simulink model "pdmRecipPump"  (R2025b)
settings: Solver=VariableStepAuto  StartTime=0.0  StopTime=2  RelTol=1e-3  EnableMultiTasking=on
values from neighbouring files (symbols this model uses):
  s = load(dataFile)    [run_0.m]    (also in run_1.m; run_2.m; run_3.m; run_4.m)
undefined symbols (not defined in the file or in its folder): bearing_fault_frict_WKSP, bearing_visc_frict_WKSP, noise_seed_offset_WKSP, smiData, TRP_Par, X, Y, Z
libraries: sm_lib x41, fl_lib x23, nesl_utility x9, simulink x7, SimscapeFluids_lib x4, sm_pump_triplex_lib x3, ee_lib x2, Mech_Hydro_Elec_Multibody_Lib x1
(part 1 of 2)
CloseFcn:
  | try,close(h1_sm_pump_triplex),end
  | clear h1_sm_pump_triplex
  | try,close(h2_sm_pump_triplex),end
  | clear h2_sm_pump_triplex
  | try,close(h3_sm_pump_triplex),end
  | clear h3_sm_pump_triplex
  | try,close(h4_sm_pump_triplex),end
  | clear h4_sm_pump_triplex
  | try,close(h5_sm_pump_triplex),end
  | clear h5_sm_pump_triplex
  | try,close(h6_sm_pump_triplex),end
  | clear h6_sm_pump_triplex
  | try,close(h7_sm_pump_triplex),end
  | clear h7_sm_pump_triplex
  | 
  | clear simlog_sm_pump_triplex
  | clear logsout_sm_pump_triplex
Description:
  | Triplex Pump with Faults
settings Model: SimulationMode=accelerator  Creator=The MathWorks, Inc.  LastModifiedBy=The MathWorks, Inc.
settings SolverCC: MaxConsecutiveMinStep=10  AlgebraicLoopSolver=TrustRegion
settings DataIOCC: InitialState=sm_pump_triplex_xFinal_steady_no_fault  LimitDataPoints=on  MaxDataPoints=10000  SignalLoggingName=logsout_sm_pump_triplex
settings OptimizationCC: LifeSpan=inf
settings DebuggingCC: AlgebraicLoopMsg=error  UnconnectedInputMsg=warning  UnconnectedOutputMsg=warning  UnconnectedLineMsg=warning  AllowSymbolicDim=off  SFUnexpectedBacktrackingDiag=warning  SFNoUnconditionalDefaultTransitionDiag=warning  SFExecutionAtInitializationDiag=none  ArithmeticOperatorsInVariantConditions=warning
settings ModelReferenceCC: EnableRefExpFcnMdlSchedulingChecks=on
settings SFSimCC: SimUseLocalCustomCode=off  CustomCodeUndefinedFunction=UseInterfaceOnly
settings RTWCC: RTWUseLocalCustomCode=off  GPUComputeCapability=3.5
settings CodeAppCC: StateflowObjectComments=on
settings GRTTargetCC: TargetLangStandard=C89/C90 (ANSI)
settings ConfigComp: CovMetricSettings=dw  CovSaveCumulativeToWorkspaceVar=on  CovSaveSingleToWorkspaceVar=on  CovExternalEMLEnable=off  CovSFcnEnable=off
settings SimscapeCC: SimscapeNominalValues="[{\"value\":\"10\",\"unit\":\"V\"},{\"value\":\"1\",\"unit\":\"A\"},{\"value\":\"10\",\"unit\":\"N*m\"},{\"value\":\"10\",\"unit\":\"bar\"},{\"value\":\"100\",\"unit\":\"kJ/kg\"},{\"value\":\"1\",\"unit\":\"kW\"},{\"value\":\"300\",\"unit\":\"K\"},{\"value\":\"100\",\"unit\":\"cm^3/s\"},{\"value\":\"1\",\"unit\":\"kN\"},{\"value\":\"1\",\"unit\":\"g/cm^3\"},{\"value\":\"1\",\"unit\":\"l\"},{\"value\":\"1\",\"unit\":\"cm^2\"},{\"value\":\"60\",\"unit\":\"Hz\"}]"  SimscapeLogType=all  SimscapeLogSimulationStatistics=on  SimscapeLogName=simlog_sm_pump_triplex  SimscapeLogDataHistory=20000.0  SimscapeOperatingPoint=sm_pump_triplex_op_steady_no_fault
settings ConfigurationSet: Description=SimMechanics 2G
settings DiagnosticsConfigSet: SimMechanicsUnsatisfiedHighPriorityTargets=none
settings ExplorerConfigSet: SimMechanicsOpenEditorOnUpdate=off  InternalSimMechanicsExplorerSettings="<ExplorerConfiguration><canonicalview>default</canonicalview><AnimationSetting><BasePlaybackSpeed>1.0</BasePlaybackSpeed><PlaybackSpeedFactor>0.0625</PlaybackSpeedFactor></AnimationSetting><TilePanel><TileInfo><Tiles Columns=\"1\" Count=\"1\" Rows=\"1\"><Column Weight=\"1\"/><Row Weight=\"1\"/><Tile Height=\"1\" Width=\"1\" X=\"0\" Y=\"0\"/></Tiles></TileInfo><SceneInfo><SceneViewer><BGColor><R>1</R><G>1</G><B>1</B></BGColor><Camera><DoPerspective>off</DoPerspective><Position><X>0.7191096199114555</X><Y>0.503364840615347475</Y><Z>-0.352088882323819574</Z></Position><Center><X>-0.0103509884654966189</X><Y>-0.00162371159480596133</Y><Z>0.10929358696063457</Z></Center><Up><X>-0.420672049294932404</X><Y>0.863070110116374023</Y><Z>0.279544293387851028</Z></Up><ViewLimDist>1</ViewLimDist><YLim>0.161872532968254601</YLim><XLim>0.255851100680109855</XLim></Camera></SceneViewer></SceneInfo></TilePanel><MechEditorPanel><Cameras/><GfxPanelCameraMap/><VideoCreator><PlaybackSpeedRatio>1.0</PlaybackSpeedRatio><FrameRate>30</FrameRate><VideoFormat>Motion JPEG AVI</VideoFormat><FrameSize>auto</FrameSize></VideoCreator></MechEditorPanel></ExplorerConfiguration>"

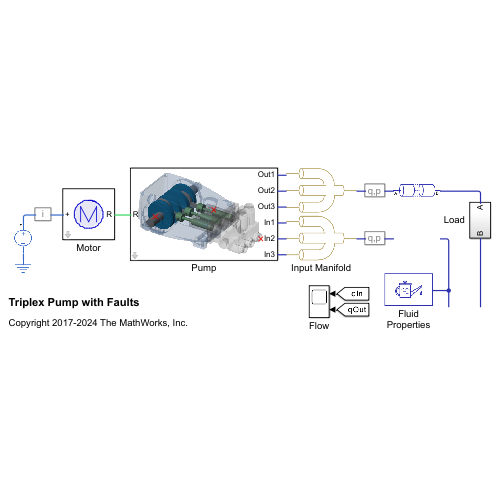
[thumbnail: Simulink's stored preview of the top-level diagram]
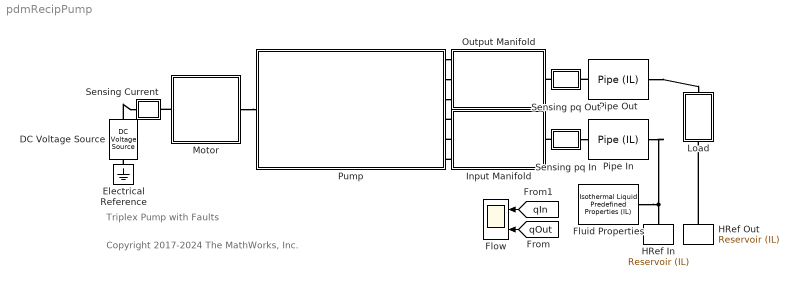
== system pdmRecipPump ==
  note: Copyright 2017-2024 The MathWorks, Inc.
  note: Triplex Pump with Faults
  DC Voltage Source : ee_lib/Additional Components/SPICE Sources/DC Voltage Source  DC=24 V
  Electrical Reference : fl_lib/Electrical/Electrical Elements/Electrical Reference
  Flow : Scope  NumInputPorts=2
      settings: ActiveDisplayYMinimum=-5.41174  ActiveDisplayYMaximum=48.70569
  Fluid Properties : SimscapeFluids_lib/Isothermal Liquid/Utilities/Isothermal Liquid Predefined Properties (IL)  fluid_list=13  concentration_param_EG=fluids.isothermal_liquid.utilities.enum.isothermal_liquid_concentration.volume_fraction  concentration_param_PG=fluids.isothermal_liquid.utilities.enum.isothermal_liquid_concentration.volume_fraction  c_mass_SW=3.5e-3  c_mass_EG=0.1  c_mass_PG=0.1  c_mass_GL=0.1  c_vol_EG=0.1  c_vol_PG=0.1  beta_L_atm_EG=2.1791 GPa  beta_L_atm_PG=2.1791 GPa  beta_L_atm_GL=2.1791 GPa  p_min_EG=0.01 MPa  p_min_PG=0.01 MPa  p_min_GL=0.01 MPa  T=60 degC  derate_coeff=1  p_atm=0.101325 MPa  properties_range_check=simscape.enum.assert.action.error  air_fraction=0.005  polytropic_index=1.0  rho_g_atm=851.6 kg/m^3  air_dissolution_model=false  p_crit=3 MPa
      settings: LibrarySourceBlock=SimscapeFluids_lib/Isothermal Liquid/Utilities/Isothermal Liquid Predefined Properties (IL)  InternalSimscapePortConfiguration="{\"Bottom\":[],\"Left\":[],\"Right\":[{\"id\":\"A\",\"label\":\"\",\"type\":\"foundation.isothermal_liquid.isothermal_liquid\"}],\"Top\":[]}"
  HRef In : fl_lib/Isothermal Liquid/Elements/Reservoir (IL)  reservoir_type=foundation.enum.constant_controlled.constant  pressure_spec=foundation.enum.pressure_spec.atmospheric  reservoir_pressure=0.101325 MPa
  HRef Out : fl_lib/Isothermal Liquid/Elements/Reservoir (IL)  reservoir_type=foundation.enum.constant_controlled.constant  pressure_spec=foundation.enum.pressure_spec.atmospheric  reservoir_pressure=0.101325 MPa
  Input Manifold : Subsystem
      mask Display: image('sm_pump_triplex_Manifold_IMAGE.png');
  Load : Subsystem
  Motor : Subsystem  Tag=PublishSubsystem  VariantControl=Electric  mask(Motor and Motor Driver){winding_fault_enable=Off}
      mask prompts: winding_fault_enable "Winding Fault"
      mask help: Model abstracts the torque-speed behavior of the combined motor and motor driver. Electric and control parameters are specified on blocks within the subsystem. The winding fault modelsa broken winding. When enabled, motor torque is set to 0 when the shaft angle is between 240 and 360 degrees (one-third of a shaft rotation).
      mask TypeOptions winding_fault_enable: Off | On
      mask Display:
      | % Circle
      | patch(sin(0:0.1:2.2*pi)*0.80,cos(0:0.1:2.2*pi)*0.80,[0.9 0.9 0.97]);
      | color('blue');
      | plot(sin(0:0.1:2.2*pi)*0.9,cos(0:0.1:2.2*pi)*0.9);
      | 
      | % 'M'
      | plot([0.5 0.5],[-0.5 0.5]);
      | plot([-0.5 -0.5],[-0.5 0.5]);
      | plot([0.5 0],[0.5 -0.5]);
      | plot([-0.5 0],[0.5 -0.5]);
      | 
      | color('red');
      | if(strcmp(get_param(gcb,'winding_fault_enable'),'On'))
      |     plot([0.85 0.6],[1.1 0.9])
      |     plot([0.6 0.85],[1.1 0.9])
      | end
      | 
      | % Plot points to set plot range
      | color('white');plot(1.6,1.6);plot(-1.6,-1.6)
      | color('black');
  Output Manifold : Subsystem
      mask Display: image('sm_pump_triplex_Manifold_IMAGE.png');
  Pipe In : SimscapeFluids_lib/Isothermal Liquid/Pipes & Fittings/Pipe (IL)  dynamic_compressibility=true  inertia=false  num_segments=1  pipe_length=5 m  cross_section_geometry=fluids.isothermal_liquid.pipes_fittings.enum.cross_section_geometry.circular  pipe_diameter=0.03 m  pipe_inner_diameter=0.05 m  pipe_outer_diameter=0.1 m  pipe_width=0.1 m  pipe_height=0.1 m  pipe_major_axis=0.1 m  pipe_minor_axis=0.05 m  pipe_side=0.1 m  pipe_angle=30 deg  pipe_area=1e-4 m^2  Dh=1.12e-2 m  elevation_spec=foundation.enum.constant_variable.constant  elevation_gain=0 m  gravity_spec=foundation.enum.constant_variable.constant  g=9.81 m/s^2  pressure_loss_spec=fluids.isothermal_liquid.pipes_fittings.enum.pressure_loss_spec.haaland  mdot_nominal=[.1, 1] kg/s  p_diff_nominal=[.001, .01] MPa  mdot_threshold=1e-6 kg/s  local_pressure_loss_spec=fluids.isothermal_liquid.pipes_fittings.enum.local_loss_spec.aggregate_length  length_add=1 m  loss_coefficient=0.1  roughness_spec=fluids.isothermal_liquid.pipes_fittings.enum.roughness_spec.custom  roughness=15e-6 m  Re_friction_TLU=[400, 1000, 1500, 3000, 4000, 6000, 10000, 20000, 40000, 60000, 100000, 100000000]  friction_factor_TLU=[.264, .112, .071, .0417, .0387, .0268, .025, .0232, .0226, .022, .0214, .0214]  Re_lam=2000  Re_tur=4000  shape_factor=64  pipe_wall_spec=fluids.isothermal_liquid.pipes_fittings.enum.wall_spec.rigid  vol_expansion_spec=fluids.isothermal_liquid.pipes_fittings.enum.vol_expansion_spec.area  area_pressure_gain=1e-6 m^2/MPa  static_pressure_TLU=[.1, 1] MPa  area_pressure_gain_TLU=[1e-05, 1.1e-05] m^2  material_behavior_spec=fluids.isothermal_liquid.pipes_fittings.enum.PipeMaterialBehavior.Linear  diameter_pressure_gain=2e-12 m/Pa  wall_thickness=0.05 m  elastic_modulus=69 GPa  stress_TLU=[276, 310] MPa  strain_TLU=[.004, .02]  stress_assert_action=simscape.enum.assert.action.none  stress_max=400 MPa  poisson_ratio=0.33  wall_time_constant=0.01 s  p0=0 + 101325 Pa  mdot0=0 kg/s
      settings: InternalSimscapePortConfiguration="{\"Bottom\":[],\"Left\":[{\"id\":\"A\",\"label\":\"A\",\"type\":\"foundation.isothermal_liquid.isothermal_liquid\"}],\"Right\":[{\"id\":\"B\",\"label\":\"B\",\"type\":\"foundation.isothermal_liquid.isothermal_liquid\"}],\"Top\":[]}"
  Pipe Out : SimscapeFluids_lib/Isothermal Liquid/Pipes & Fittings/Pipe (IL)  dynamic_compressibility=true  inertia=false  num_segments=1  pipe_length=5 m  cross_section_geometry=fluids.isothermal_liquid.pipes_fittings.enum.cross_section_geometry.circular  pipe_diameter=0.03 m  pipe_inner_diameter=0.05 m  pipe_outer_diameter=0.1 m  pipe_width=0.1 m  pipe_height=0.1 m  pipe_major_axis=0.1 m  pipe_minor_axis=0.05 m  pipe_side=0.1 m  pipe_angle=30 deg  pipe_area=1e-4 m^2  Dh=1.12e-2 m  elevation_spec=foundation.enum.constant_variable.constant  elevation_gain=0 m  gravity_spec=foundation.enum.constant_variable.constant  g=9.81 m/s^2  pressure_loss_spec=fluids.isothermal_liquid.pipes_fittings.enum.pressure_loss_spec.haaland  mdot_nominal=[.1, 1] kg/s  p_diff_nominal=[.001, .01] MPa  mdot_threshold=1e-6 kg/s  local_pressure_loss_spec=fluids.isothermal_liquid.pipes_fittings.enum.local_loss_spec.aggregate_length  length_add=1 m  loss_coefficient=0.1  roughness_spec=fluids.isothermal_liquid.pipes_fittings.enum.roughness_spec.custom  roughness=15e-6 m  Re_friction_TLU=[400, 1000, 1500, 3000, 4000, 6000, 10000, 20000, 40000, 60000, 100000, 100000000]  friction_factor_TLU=[.264, .112, .071, .0417, .0387, .0268, .025, .0232, .0226, .022, .0214, .0214]  Re_lam=2000  Re_tur=4000  shape_factor=64  pipe_wall_spec=fluids.isothermal_liquid.pipes_fittings.enum.wall_spec.rigid  vol_expansion_spec=fluids.isothermal_liquid.pipes_fittings.enum.vol_expansion_spec.area  area_pressure_gain=1e-6 m^2/MPa  static_pressure_TLU=[.1, 1] MPa  area_pressure_gain_TLU=[1e-05, 1.1e-05] m^2  material_behavior_spec=fluids.isothermal_liquid.pipes_fittings.enum.PipeMaterialBehavior.Linear  diameter_pressure_gain=2e-12 m/Pa  wall_thickness=0.05 m  elastic_modulus=69 GPa  stress_TLU=[276, 310] MPa  strain_TLU=[.004, .02]  stress_assert_action=simscape.enum.assert.action.none  stress_max=400 MPa  poisson_ratio=0.33  wall_time_constant=0.01 s  p0=TRP_Par.Spec.p_output + 1.01325 bar  mdot0=0 kg/s
      settings: InternalSimscapePortConfiguration="{\"Bottom\":[],\"Left\":[{\"id\":\"A\",\"label\":\"A\",\"type\":\"foundation.isothermal_liquid.isothermal_liquid\"}],\"Right\":[{\"id\":\"B\",\"label\":\"B\",\"type\":\"foundation.isothermal_liquid.isothermal_liquid\"}],\"Top\":[]}"
  Pump : Subsystem  Tag=PublishSubsystem  mask(Triplex Pump with Faults){cyl_gap_P=TRP_Par.Cylinder.gap, cyl_rad_out_P=TRP_Par.Cylinder.rad_outer, cyl_len_P=TRP_Par.Cylinder.len, cyl_stroke_P=TRP_Par.Cylinder.stroke, cyl_frict_brkway_frc_P=TRP_Par.Cylinder.Friction.BrkFrc, cyl_frict_brkway_vel_P=TRP_Par.Cylinder.Friction.BrkVel, cyl_frict_col_frc_P=TRP_Par.Cylinder.Friction.ColFrc, cyl_frict_visc_coef_P=TRP_Par.Cylinder.Friction.ViscCo, cyl_rho_P=TRP_Par.Cylinder.rho, cyl_clr_P=TRP_Par.Cylinder.clr, cyl_opc_P=TRP_Par.Cylinder.opc, plgB_len_P=TRP_Par.Plunger.len, plgB_rad_P=TRP_Par.Plunger.rad, stem_len_P=TRP_Par.Stem.len, stem_rad_P=TRP_Par.Stem.rad, pin_len_P=TRP_Par.Pin.len, pin_rad_P=TRP_Par.Pin.rad, cup_rad_out_P=TRP_Par.StemCup.rad, cup_thk_P=TRP_Par.StemCup.wall, cup_len_P=TRP_Par.StemCup.len, cup_pinOffset_P=TRP_Par.StemCup.pinOffset, plg_rho_P=TRP_Par.Plunger.rho, plg_clr_P=TRP_Par.Plunger.clr, plg_opc_P=TRP_Par.Plunger.opc, conrod_len_P=TRP_Par.ConRod.len, conrod_web_widP_P=TRP_Par.ConRod.W1, conrod_web_widC_P=TRP_Par.ConRod.W2, conrod_ringC_wid_P=TRP_Par.ConRod.R2.width, conrod_ringP_wid_P=TRP_Par.ConRod.R1.width, crank_shaft_rad_P=TRP_Par.Crank.Shaft.rad, conrod_thk_P=TRP_Par.ConRod.hei, conrod_rho_P=TRP_Par.ConRod.rho, conrod_clr_P=TRP_Par.ConRod.clr, conrod_opc_P=TRP_Par.ConRod.opc, chkv_in_maxA_P=TRP_Par.Check_Valve.In.Max_Area, chkv_out_maxA_P=TRP_Par.Check_Valve.Out.Max_Area, chkv_in_crkP_P=TRP_Par.Check_Valve.In.Crack_Pr, chkv_out_crkP_P=TRP_Par.Check_Valve.Out.Crack_Pr, chkv_in_maxOpenP_P=TRP_Par.Check_Valve.In.Max_Open_Pr, chkv_out_maxOpenP_P=TRP_Par.Check_Valve.Out.Max_Open_Pr, chkv_vis_popup_P=Off, chkv_vis_rad_in_P=TRP_Par.Check_Valve.In.Vis.rad, chkv_vis_rad_out_P=TRP_Par.Check_Valve.Out.Vis.rad, chkv_vis_clr_in_P=TRP_Par.Check_Valve.In.Vis.clr, chkv_vis_clr_out_P=TRP_Par.Check_Valve.Out.Vis.clr, shaft_rad_P=TRP_Par.Crank.Shaft.rad, shaft_len_P=TRP_Par.Crank.Shaft.len, web_rad_P=TRP_Par.Crank.Cam.rad, web_len_P=TRP_Par.Crank.Cam.wid, motor_shaft_rad_P=TRP_Par.Motor.Shaft.rad, motor_shaft_len_P=TRP_Par.Motor.Shaft.len, shaft_pos_P=TRP_Par.Crank.Shaft.pos, crank_rho_P=TRP_Par.Crank.rho, bearing_visc_frict=TRP_Par.Crank.Bearing.b, crank_clr_P=TRP_Par.Crank.Cam.clr, motor_shaft_clr_P=TRP_Par.Motor.Shaft.clr, crank_opc_P=TRP_Par.Crank.Cam.opc, crank_ax_offset=TRP_Par.Crank.axoffset, bearing_sep=TRP_Par.Crank.Bearing_sep, housing_clr=TRP_Par.Housing.clr, housing_opc=TRP_Par.Housing.opc, manifold_clr=TRP_Par.Manifold.clr, manifold_opc=TRP_Par.Manifold.opc, leak_cyl1_popup=On, Run Time, leak_cyl2_popup=Off, leak_cyl3_popup=Off, leak_cyl1_area=TRP_Par.Check_Valve.In.Max_Area*0.05, leak_cyl2_area=TRP_Par.Check_Valve.In.Max_Area*0.05, leak_cyl3_area=TRP_Par.Check_Valve.In.Max_Area*0.05, block_in_cyl1_popup=On, Run Time, block_in_cyl2_popup=Off, block_in_cyl3_popup=Off, block_in_cyl1_factor=0.5, block_in_cyl2_factor=0.5, block_in_cyl3_factor=0.5, bearing_fault_popup=On, Run Time, bearing_fault_frict=3e-4, seal_leak_vis_len_P=TRP_Par.Seal_Leak.len, seal_leak_vis_rad_P=TRP_Par.Seal_Leak.rad, seal_leak_vis_clr_P=TRP_Par.Seal_Leak.clr, inlet_obstr_len_P=TRP_Par.Manifold.Inlet.obstr.len, inlet_obstr_rad_P=TRP_Par.Manifold.Inlet.rad, inlet_obstr_clr_P=TRP_Par.Manifold.Inlet.obstr.clr, bearing_fault_vis_len=TRP_Par.Crank.Bearing_Fault.len, bearing_fault_vis_rad=TRP_Par.Crank.Bearing_Fault.rad, bearing_fault_vis_clr=TRP_Par.Crank.Bearing_Fault.clr, bearing_fault_vis_opc=0}
      mask prompts: cyl_gap_P "Gap (m)"; cyl_rad_out_P "Outer Radius (m)"; cyl_len_P "Length (m)"; cyl_stroke_P "Stroke (m)"; cyl_frict_brkway_frc_P "Breakaway Friction Force (N)"; cyl_frict_brkway_vel_P "Breakaway Friction Velocity (m/s)"; cyl_frict_col_frc_P "Coulomb Friction Force (N)"; cyl_frict_visc_coef_P "Viscous Friction Coeff (N/(m/s))"; cyl_rho_P "Density (kg/m^3)"; cyl_clr_P "Color [RGB]"; cyl_opc_P "Opacity (0-1)"; cup_rad_out_P "Outer Radius (m)"; cup_thk_P "Wall Thickness (m)"; cup_len_P "Length(m)"; cup_pinOffset_P "Pin Offset (m)"; plg_rho_P "Density (kg/m^3)"; plg_clr_P "Color [RGB]"; plg_opc_P "Opacity (0-1)"; conrod_len_P "Length, center-center (m)"; conrod_web_widP_P "Width, pin end (m)"; conrod_web_widC_P "Width, crank end (m)"; conrod_ringC_wid_P "Crank Ring Width (m)"; conrod_ringP_wid_P "Pin Ring Width (m)"; crank_shaft_rad_P "Crank Shaft Radius (m)"; conrod_thk_P "Thickness (m)"; conrod_rho_P "Density (kg/m^3)"; conrod_clr_P "Color [RGB]"; conrod_opc_P "Opacity (0-1)"; chkv_vis_popup_P "Valve Visualization"; shaft_pos_P "Crankpin Axis Offset (m)"; crank_rho_P "Density (kg/m^3)"; bearing_visc_frict "Bearing Viscous Friction (N*m/(deg/s))"; crank_clr_P "Crank Color [RGB]"; motor_shaft_clr_P "Motor Shaft Color [RGB]"; crank_opc_P "Opacity (0-1)"; crank_ax_offset "Crankshaft Axis Offset [XYZ] (m)"; bearing_sep "Bearing Separation (m)"; housing_clr "Housing Color [RGB]"; housing_opc "Housing Opacity (0-1)"; manifold_clr "Manifold Color [RGB]"; manifold_opc "Manifold Opacity (0-1)"; leak_cyl1_area "Plunger 1 Leak Area (m^2)"; leak_cyl2_area "Plunger 2 Leak Area (m^2)"; leak_cyl3_area "Plunger 3 Leak Area (m^2)"; block_in_cyl1_factor "Blocked Inlet 1: Area Factor (0-1)"; block_in_cyl2_factor "Blocked Inlet 2: Area Factor (0-1)"; block_in_cyl3_factor "Blocked Inlet 3: Area Factor (0-1)"; bearing_fault_popup "Bearing Wear"; bearing_fault_frict "Additional Friction (N*m/(deg/s))"; seal_leak_vis_len_P "Length (m)"; seal_leak_vis_rad_P "Radius (m)"; seal_leak_vis_clr_P "Color [RGB]"; inlet_obstr_len_P "Length (m)"; inlet_obstr_rad_P "Radius (m)"; inlet_obstr_clr_P "Color [RGB]"; bearing_fault_vis_len "Length (m)"; bearing_fault_vis_rad "Radius (m)"; bearing_fault_vis_clr "Color [RGB]"; bearing_fault_vis_opc "Opacity (0-1)"
      mask help: Models a triplex pump. Three hydraulic plungers are connected to a crankshaft. Hydraulic and mechanical faults can be enabled on the Faults tab.
      mask init:
      | % -- Configure Plunger Faults
      | set_param([gcb '/Plunger 1'],'leak_cyl_popup',...
      |     get_param(gcb,'leak_cyl1_popup'));
      | set_param([gcb '/Plunger 2'],'leak_cyl_popup',...
      |     get_param(gcb,'leak_cyl2_popup'));
      | set_param([gcb '/Plunger 3'],'leak_cyl_popup',...
      |     get_param(gcb,'leak_cyl3_popup'));
      | 
      | set_param([gcb '/Plunger 1'],'block_in_popup',...
      |     get_param(gcb,'block_in_cyl1_popup'));
      | set_param([gcb '/Plunger 2'],'block_in_popup',...
      |     get_param(gcb,'block_in_cyl2_popup'));
      | set_param([gcb '/Plunger 3'],'block_in_popup',...
      |     get_param(gcb,'block_in_cyl3_popup'));
      | 
      | % -- Set valve visualization
      | set_param([gcb '/Plunger 1'],'chkv_vis_popup',...
      |     get_param(gcb,'chkv_vis_popup_P'));
      | set_param([gcb '/Plunger 2'],'chkv_vis_popup',...
      |     get_param(gcb,'chkv_vis_popup_P'));
      | set_param([gcb '/Plunger 3'],'chkv_vis_popup',...
      |     get_param(gcb,'chkv_vis_popup_P'));
      | 
      | % -- Configure bearing fault
      | if(bearing_fault_popup==1)
      |     set_param([gcb '/Revolute Crank'],...
      |         'DampingCoefficient','bearing_visc_frict',...
      |         'DampingCoefficient_conf','compiletime');
      |     bearing_fault_vis_opc = 0;
      | elseif(bearing_fault_popup==2)
      |     set_param([gcb '/Revolute Crank'],...
      |         'DampingCoefficient','bearing_visc_frict+bearing_fault_frict',...
      |         'DampingCoefficient_conf','compiletime');
      |     bearing_fault_vis_opc = 1;
      | elseif(bearing_fault_popup==3)
      |     set_param([gcb '/Revolute Crank'],...
      |         'DampingCoefficient','bearing_visc_frict_WKSP+bearing_fault_frict_WKSP',...
      |         'DampingCoefficient_conf','runtime');
      |     bearing_fault_vis_opc = 1;
      | end
      mask TypeOptions chkv_vis_popup_P: Off | On
      mask TypeOptions leak_cyl1_popup: Off | On | On, Run Time
      mask Callback leak_cyl1_popup:
      | maskObj = Simulink.Mask.get(gcb);
      | leak_cyl1_area_h = maskObj.getParameter('leak_cyl1_area');
      | leak_cyl1_text_h = maskObj.getDialogControl('leak_cyl1_tune_text');
      | if (strcmp(get_param(gcb,'leak_cyl1_popup'),'Off'))
      |     leak_cyl1_area_h.Visible = 'off';
      |     leak_cyl1_text_h.Visible = 'off';
      | elseif (strcmp(get_param(gcb,'leak_cyl1_popup'),'On'))
      |     leak_cyl1_area_h.Visible = 'on';
      |     leak_cyl1_text_h.Visible = 'off';
      | elseif (strcmp(get_param(gcb,'leak_cyl1_popup'),'On, Run Time'))
      |     leak_cyl1_area_h.Visible = 'off';
      |     leak_cyl1_text_h.Visible = 'on';
      | end
      | clear maskObj leak_cyl1_area_h leak_cyl1_text_h
      mask TypeOptions leak_cyl2_popup: Off | On | On, Run Time
      mask Callback leak_cyl2_popup:
      | maskObj = Simulink.Mask.get(gcb);
      | leak_cyl2_area_h = maskObj.getParameter('leak_cyl2_area');
      | leak_cyl2_text_h = maskObj.getDialogControl('leak_cyl2_tune_text');
      | if (strcmp(get_param(gcb,'leak_cyl2_popup'),'Off'))
      |     leak_cyl2_area_h.Visible = 'off';
      |     leak_cyl2_text_h.Visible = 'off';
      | elseif (strcmp(get_param(gcb,'leak_cyl2_popup'),'On'))
      |     leak_cyl2_area_h.Visible = 'on';
      |     leak_cyl2_text_h.Visible = 'off';
      | elseif (strcmp(get_param(gcb,'leak_cyl2_popup'),'On, Run Time'))
      |     leak_cyl2_area_h.Visible = 'off';
      |     leak_cyl2_text_h.Visible = 'on';
      | end
      | clear maskObj leak_cyl2_area_h leak_cyl2_text_h
      mask TypeOptions leak_cyl3_popup: Off | On | On, Run Time
      mask Callback leak_cyl3_popup:
      | maskObj = Simulink.Mask.get(gcb);
      | leak_cyl3_area_h = maskObj.getParameter('leak_cyl3_area');
      | leak_cyl3_text_h = maskObj.getDialogControl('leak_cyl3_tune_text');
      | if (strcmp(get_param(gcb,'leak_cyl3_popup'),'Off'))
      |     leak_cyl3_area_h.Visible = 'off';
      |     leak_cyl3_text_h.Visible = 'off';
      | elseif (strcmp(get_param(gcb,'leak_cyl3_popup'),'On'))
      |     leak_cyl3_area_h.Visible = 'on';
      |     leak_cyl3_text_h.Visible = 'off';
      | elseif (strcmp(get_param(gcb,'leak_cyl3_popup'),'On, Run Time'))
      |     leak_cyl3_area_h.Visible = 'off';
      |     leak_cyl3_text_h.Visible = 'on';
      | end
      | clear maskObj leak_cyl3_area_h leak_cyl3_text_h
      mask TypeOptions block_in_cyl1_popup: Off | On | On, Run Time
      mask Callback block_in_cyl1_popup:
      | maskObj = Simulink.Mask.get(gcb);
      | cyl_factor_h = maskObj.getParameter('block_in_cyl1_factor');
      | cyl_text_h = maskObj.getDialogControl('block_in_cyl1_tune_text');
      | tmp_block_in_cyl = get_param(gcb,'block_in_cyl1_popup');
      | 
      | if (strcmp(tmp_block_in_cyl,'Off'))
      |     cyl_factor_h.Visible = 'off';
      |     cyl_text_h.Visible = 'off';
      | elseif (strcmp(tmp_block_in_cyl,'On'))
      |     cyl_factor_h.Visible = 'on';
      |     cyl_text_h.Visible = 'off';
      | elseif (strcmp(tmp_block_in_cyl,'On, Run Time'))
      |     cyl_factor_h.Visible = 'off';
      |     cyl_text_h.Visible = 'on';
      | end
      | clear maskObj tmp_block_in_cyl cyl_factor_h cyl_text_h
      mask TypeOptions block_in_cyl2_popup: Off | On | On, Run Time
      mask Callback block_in_cyl2_popup:
      | maskObj = Simulink.Mask.get(gcb);
      | cyl_factor_h = maskObj.getParameter('block_in_cyl2_factor');
      | cyl_text_h = maskObj.getDialogControl('block_in_cyl2_tune_text');
      | tmp_block_in_cyl = get_param(gcb,'block_in_cyl2_popup');
      | 
      | if (strcmp(tmp_block_in_cyl,'Off'))
      |     cyl_factor_h.Visible = 'off';
      |     cyl_text_h.Visible = 'off';
      | elseif (strcmp(tmp_block_in_cyl,'On'))
      |     cyl_factor_h.Visible = 'on';
      |     cyl_text_h.Visible = 'off';
      | elseif (strcmp(tmp_block_in_cyl,'On, Run Time'))
      |     cyl_factor_h.Visible = 'off';
      |     cyl_text_h.Visible = 'on';
      | end
      | clear maskObj tmp_block_in_cyl cyl_factor_h cyl_text_h
      mask TypeOptions block_in_cyl3_popup: Off | On | On, Run Time
      mask Callback block_in_cyl3_popup:
      | maskObj = Simulink.Mask.get(gcb);
      | cyl_factor_h = maskObj.getParameter('block_in_cyl3_factor');
      | cyl_text_h = maskObj.getDialogControl('block_in_cyl3_tune_text');
      | tmp_block_in_cyl = get_param(gcb,'block_in_cyl3_popup');
      | 
      | if (strcmp(tmp_block_in_cyl,'Off'))
      |     cyl_factor_h.Visible = 'off';
      |     cyl_text_h.Visible = 'off';
      | elseif (strcmp(tmp_block_in_cyl,'On'))
      |     cyl_factor_h.Visible = 'on';
      |     cyl_text_h.Visible = 'off';
      | elseif (strcmp(tmp_block_in_cyl,'On, Run Time'))
      |     cyl_factor_h.Visible = 'off';
      |     cyl_text_h.Visible = 'on';
      | end
      | clear maskObj tmp_block_in_cyl cyl_factor_h cyl_text_h
      mask TypeOptions bearing_fault_popup: Off | On | On, Run Time
      mask Callback bearing_fault_popup:
      | maskObj = Simulink.Mask.get(gcb);
      | bf_frict_h = maskObj.getParameter('bearing_fault_frict');
      | bf_text_h = maskObj.getDialogControl('bearing_fault_tune_text');
      | tmp_bearing_fault = get_param(gcb,'bearing_fault_popup');
      | 
      | if (strcmp(tmp_bearing_fault,'Off'))
      |     bf_frict_h.Visible = 'off';
      |     bf_text_h.Visible = 'off';
      | elseif (strcmp(tmp_bearing_fault,'On'))
      |     bf_frict_h.Visible = 'on';
      |     bf_text_h.Visible = 'off';
      | elseif (strcmp(tmp_bearing_fault,'On, Run Time'))
      |     bf_frict_h.Visible = 'off';
      |     bf_text_h.Visible = 'on';
      | end
      | clear maskObj tmp_bearing_fault bf_frict_h bf_text_h
      mask DialogControl tab_cylinder Prompt: Cyl.
      mask DialogControl cont_dims Prompt: Dimensions
      mask DialogControl cont_friction Prompt: Friction
      mask DialogControl cont_cyl_vis Prompt: Cylinder Visualization
      mask DialogControl tab_plunger Prompt: Plung.
      mask DialogControl text_length Prompt: Length (m)
      mask DialogControl text_radius Prompt: Radius (m)
      mask DialogControl text_base Prompt: Base
      mask DialogControl text_stem Prompt: Stem
      mask DialogControl text_pin Prompt: Pin
      mask DialogControl cont_cup Prompt: Cup
      mask DialogControl cont_plg_vis Prompt: Plunger Visualization
      mask DialogControl tab_conrod Prompt: Rod
      mask DialogControl cont_conrodWeb Prompt: Web
      mask DialogControl cont_conrodRings Prompt: Rings
      mask DialogControl cont_conrod_vis Prompt: Rod Visualization
      mask DialogControl tab_valves Prompt: Valve
      mask DialogControl text_open_inlet Prompt: Inlet
      mask DialogControl text_open_outlet Prompt: Outlet
      mask DialogControl text_open_maxA Prompt: Max Area (m)
      mask DialogControl text_open_crkP Prompt: Crack. Pr (Pa)
      mask DialogControl text_open_maxOpenP Prompt: Max Pr. (Pa)
      mask DialogControl Container22 Prompt: Visualization Settings
      mask DialogControl text_valvis_inlet Prompt: Inlet
      mask DialogControl text_valvis_outlet Prompt: Outlet
      mask DialogControl text_valvis_rad Prompt: Radius (m)
      mask DialogControl text_valvis_clr Prompt: Color [RGB]
      mask DialogControl tab_crank Prompt: Crank
      mask DialogControl text_crank_rad Prompt: Radius (m)
      mask DialogControl text_crank_len Prompt: Length (m)
      mask DialogControl text_crankpin Prompt: Crankpin
      mask DialogControl text_web Prompt: Web
      mask DialogControl text_motor_shaft Prompt: Motor Shaft
      mask DialogControl cont_crank_vis Prompt: Crankshaft Visualization
      mask DialogControl tab_housing Prompt: Housing
      mask DialogControl cont_vis Prompt: Visualization
      mask DialogControl tab_faults Prompt: Fault
      mask DialogControl Control12 Prompt: Plunger 1
      mask DialogControl Control13 Prompt: Plunger 2
      mask DialogControl Control14 Prompt: Plunger 3
      mask DialogControl Control10 Prompt: Seal Leak
      mask DialogControl leak_cyl1_tune_text Prompt: Plunger 1:  Set >> leak_cyl_area_WKSP
      mask DialogControl leak_cyl2_tune_text Prompt: Plunger 2:  Set >> leak_cyl_area_WKSP
      mask DialogControl leak_cyl3_tune_text Prompt: Plunger 3:  Set >> leak_cyl_area_WKSP
      mask DialogControl Control19 Prompt: Blocked Inlet
      mask DialogControl block_in_cyl1_tune_text Prompt: Plunger 1: Set >> block_in_factor_WKSP, chkv_out_maxA_WKSP
      mask DialogControl block_in_cyl2_tune_text Prompt: Plunger 2: Set >> block_in_factor_WKSP, chkv_out_maxA_WKSP
      mask DialogControl block_in_cyl3_tune_text Prompt: Plunger 3: Set >> block_in_factor_WKSP, chkv_out_maxA_WKSP
      mask DialogControl bearing_fault_tune_text Prompt: Set >> bearing_visc_frict_WKSP, bearing_fault_frict_WKSP
      mask DialogControl cont_seal_leak_vis Prompt: Seal Leak Visualization
      mask DialogControl cont_blocked_line_vis Prompt: Blocked Line Visualization
      mask DialogControl cont_bearing_fault_vis Prompt: Bearing Fault Visualization
      mask Display:
      | image('sm_pump_triplex_Pump_IMAGE.png');
      | color('white');
      | plot(0,0);
      | plot(659,412);
      | color('red');
      | if(~strcmp(get_param(gcb,'block_in_cyl3_popup'),'Off'))
      |     plot([510 530],[30 50]);
      |     plot([530 510],[30 50]);
      | end
      | if(~strcmp(get_param(gcb,'block_in_cyl2_popup'),'Off'))
      |     plot([540 560],[55 75]);
      |     plot([560 540],[55 75]);
      | end
      | if(~strcmp(get_param(gcb,'block_in_cyl1_popup'),'Off'))
      |     plot([575 595],[85 105]);
      |     plot([595 575],[85 105]);
      | end
      | if(~strcmp(get_param(gcb,'leak_cyl3_popup'),'Off'))
      |     plot([300 320],[155 175]);
      |     plot([320 300],[155 175]);
      | end
      | if(~strcmp(get_param(gcb,'leak_cyl2_popup'),'Off'))
      |     plot([335 355],[185 205]);
      |     plot([355 335],[185 205]);
      | end
      | if(~strcmp(get_param(gcb,'leak_cyl1_popup'),'Off'))
      |     plot([365 385],[215 235]);
      |     plot([385 365],[215 235]);
      | end
      | if(~strcmp(get_param(gcb,'bearing_fault_popup'),'Off'))
      |     plot([100 120],[185 205]);
      |     plot([120 100],[185 205]);
      | end
  Sensing Current : Subsystem
      mask Display: disp('i');
  Sensing pq In : Subsystem
      mask Display: disp('q,p');
  Sensing pq Out : Subsystem
      mask Display: disp('q,p');
  wires:
  [qIn] -> Flow/1
  [qOut] -> Flow/2
  connections:
  Motor/RConn1 -- Pump/LConn1
  Input Manifold/LConn2 -- Pump/RConn5
  Input Manifold/LConn1 -- Pump/RConn4
  Input Manifold/LConn3 -- Pump/RConn6
  Pump/RConn1 -- Output Manifold/LConn1
  Pump/RConn2 -- Output Manifold/LConn2
  Pump/RConn3 -- Output Manifold/LConn3
  Sensing pq Out/LConn1 -- Output Manifold/RConn1
  DC Voltage Source/LConn1 -- Sensing Current/LConn1
  Electrical Reference/LConn1 -- DC Voltage Source/RConn1
  Motor/LConn1 -- Sensing Current/RConn1
  Pipe Out/LConn1 -- Sensing pq Out/RConn1
  Pipe Out/RConn1 -- Load/LConn1
  HRef Out/LConn1 -- Load/RConn1
  Fluid Properties/RConn1 -- Pipe In/LConn1 -- HRef In/LConn1
  Sensing pq In/RConn1 -- Input Manifold/RConn1
  Sensing pq In/LConn1 -- Pipe In/RConn1

== system pdmRecipPump/Input Manifold ==
  Chamber : fl_lib/Isothermal Liquid/Elements/Constant Volume Chamber (IL)  volume=2e-4 m^3  p_I_specify=off  p_I_priority=High  p_I=0 + 101325 Pa  p_I_nominal_specify=off  p_I_nominal_value=1  p_I_nominal_unit=Pa
      settings: LibrarySourceBlock=fl_lib/Isothermal Liquid/Elements/Constant Volume Chamber (IL)  InternalSimscapePortConfiguration="{\"Bottom\":[],\"Left\":[{\"id\":\"A\",\"label\":\"A\",\"type\":\"foundation.isothermal_liquid.isothermal_liquid\"}],\"Right\":[],\"Top\":[]}"
  A : PMIOPort  Side=Right
  B1 : PMIOPort  Port=2  Side=Left
  B2 : PMIOPort  Port=3  Side=Left
  B3 : PMIOPort  Port=4  Side=Left
  connections:
  Chamber/LConn1 -- A/RConn1 -- B1/RConn1 -- B2/RConn1 -- B3/RConn1

== system pdmRecipPump/Load ==
  Chamber : fl_lib/Isothermal Liquid/Elements/Constant Volume Chamber (IL)  volume=1e-4 m^3  p_I_specify=on  p_I_priority=High  p_I=TRP_Par.Spec.p_output + 1.01325 bar  p_I_nominal_specify=off  p_I_nominal_value=1  p_I_nominal_unit=Pa
      settings: LibrarySourceBlock=fl_lib/Isothermal Liquid/Elements/Constant Volume Chamber (IL)  InternalSimscapePortConfiguration="{\"Bottom\":[],\"Left\":[{\"id\":\"A\",\"label\":\"A\",\"type\":\"foundation.isothermal_liquid.isothermal_liquid\"}],\"Right\":[],\"Top\":[]}"
  Orifice : Subsystem
  Pressure Source : Subsystem
  A : PMIOPort  Side=Left
  B : PMIOPort  Port=2  Side=Right
  connections:
  Chamber/LConn1 -- Orifice/LConn1 -- A/RConn1
  Pressure Source/LConn1 -- Orifice/RConn1
  B/RConn1 -- Pressure Source/RConn1

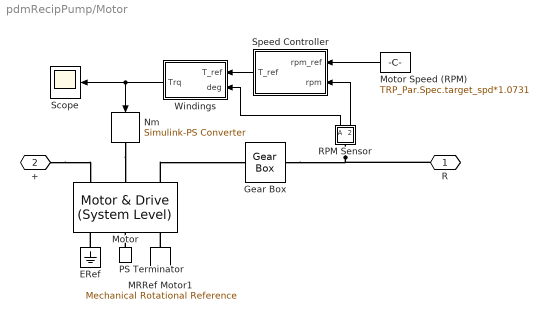
== system pdmRecipPump/Motor ==
  ERef : fl_lib/Electrical/Electrical Elements/Electrical Reference
  Gear Box : fl_lib/Mechanical/Mechanisms/Gear Box  ratio=2  t_in_specify=off  t_in_priority=None  t_in=0 N*m  t_in_nominal_specify=off  t_in_nominal_value=1  t_in_nominal_unit=N*m  t_out_specify=off  t_out_priority=None  t_out=0 N*m  t_out_nominal_specify=off  t_out_nominal_value=1  t_out_nominal_unit=N*m
  MRRef Motor1 : fl_lib/Mechanical/Rotational Elements/Mechanical Rotational Reference  Tag=Factory Generic
  Motor : ee_lib/Electromechanical/Motor & Drive (System Level)  torque_speed_param=2  overtorque_param=ee.enum.electromech.overtorque.no  T_t=[.09, .08, .07, 0] N*m  T_t_intermittent=[.36, .32, .28, 0] N*m  T_t_2D=[.09, .09, .09; .08, .08, .08; .07, .07, .07; 0, 0, 0] N*m  T_t_intermittent_2D=[.36, .36, .36; .32, .32, .32; .28, .28, .28; 0, 0, 0] N*m  w_t=[0, 3750, 7500, 8000] rpm  vdc_t=[6, 12, 24] V  torque_max=5 N*m  power_max=9000 W  torque_max_intermittent=0.4 N*m  power_max_intermittent=120 W  time_overtorque=30 s  time_recover=60 s  Tc=0.02 s  EnableSwitch=false  losses_param=1  eff=100  w_eff=958 rpm  T_eff=1 N*m  Piron=0 W  Pbase=0 W  w_eff_vec=[-8000, -4000, 0, 4000, 8000] rpm  T_eff_vec=[0, .03, .06, .09] N*m  v_eff_vec=[100, 250, 400] V  losses_mat=[1.49, 1.67, 2.21, 3.1; .42, .69, 1.14, 2.03; .06, .24, .78, 1.68; .42, .69, 1.14, 2.03; 1.49, 1.67, 2.21, 3.1] W  efficiency_mat=[95, 95, 95, 95; 95, 95, 95, 95; 95, 95, 95, 95; 95, 95, 95, 95; 95, 95, 95, 95]  losses_mat_3D=ones(5, 4, 3) W  efficiency_mat_3D=95 * ones(5, 4, 3)  Res=0 Ohm  J=5e-6*0 kg*m^2  lam=1e-5*0 N*m/(rad/s)  speed0=0 rpm  faulted_specify=off  faulted_priority=None  faulted=0  faulted_nominal_specify=off  faulted_nominal_value=1  faulted_nominal_unit=1  isSwitchedOff_specify=off  isSwitchedOff_priority=None  isSwitchedOff=0  isSwitchedOff_nominal_specify=off  isSwitchedOff_nominal_value=1  isSwitchedOff_nominal_unit=1  torqueLimitContinuous_specify=off  torqueLimitContinuous_priority=None  torqueLimitContinuous=0 N*m  torqueLimitContinuous_nominal_specify=off  torqueLimitContinuous_nominal_value=1  torqueLimitContinuous_nominal_unit=N*m  alpha=3.93e-3 1/K  Tmeas=25 degC  Tmeas2=125 degC  losses_mat_T2=[1.49, 1.74, 2.49, 3.74; .42, .67, 1.42, 2.67; .06, .31, 1.06, 2.31; .42, .67, 1.42, 2.67; 1.49, 1.74, 2.49, 3.74] W  efficiency_mat_T2=[95, 95, 95, 95; 95, 95, 95, 95; 95, 95, 95, 95; 95, 95, 95, 95; 95, 95, 95, 95]  losses_mat_3D_T2=ones(5, 4, 3) W  efficiency_mat_3D_T2=95 * ones(5, 4, 3)  thermal_mass=100 J/K  initial_temperature=25 degC
  Motor Speed (RPM) : Constant  Value=TRP_Par.Spec.target_spd*1.0731
  Nm : nesl_utility/Simulink-PS Converter  PhysicalDomain=network_engine_domain  SubClassName=ps_input  LeftPortType=input  RightPortType=output  PseudoPeriodic=off  Frequencies=[]  NoiseDistribution=none  NoiseParameters=[]  Unit=N*m  AffineConversion=off  FilteringAndDerivatives=zero  SimscapeFilterOrder=1  InputFilterTimeConstant=.001  UdotUserProvided=1
  PS Terminator : fl_lib/Physical Signals/Sinks/PS Terminator
  RPM Sensor : Subsystem
      mask Display: disp('S')
  Scope : Scope
      settings: ActiveDisplayYMinimum=-2.40087  ActiveDisplayYMaximum=21.60781
  Speed Controller : Subsystem
  Windings : Subsystem
  R : PMIOPort  Side=Right
  + : PMIOPort  Port=2  Side=Left
  wires:
  RPM Sensor/2(rpm) -> Speed Controller/2(rpm)
  Motor Speed (RPM)/1 -> Speed Controller/1(rpm_ref)
  Speed Controller/1(T_ref) -> Windings/1(T_ref)
  RPM Sensor/1(A) -> Windings/2(deg)
  Windings/1(Trq) -> Scope/1, Nm/1
  connections:
  ERef/LConn1 -- Motor/RConn1
  Nm/RConn1 -- Motor/LConn2
  PS Terminator/LConn1 -- Motor/RConn2
  +/RConn1 -- Motor/LConn1
  MRRef Motor1/LConn1 -- Motor/RConn3
  RPM Sensor/LConn1 -- Gear Box/RConn1 -- R/RConn1
  Motor/LConn3 -- Gear Box/LConn1

== system pdmRecipPump/Output Manifold ==
  Chamber : fl_lib/Isothermal Liquid/Elements/Constant Volume Chamber (IL)  volume=2e-4 m^3  p_I_specify=on  p_I_priority=High  p_I=TRP_Par.Spec.p_output + 1.01325 bar  p_I_nominal_specify=off  p_I_nominal_value=1  p_I_nominal_unit=Pa
      settings: LibrarySourceBlock=fl_lib/Isothermal Liquid/Elements/Constant Volume Chamber (IL)  InternalSimscapePortConfiguration="{\"Bottom\":[],\"Left\":[{\"id\":\"A\",\"label\":\"A\",\"type\":\"foundation.isothermal_liquid.isothermal_liquid\"}],\"Right\":[],\"Top\":[]}"
  B : PMIOPort  Side=Right
  A1 : PMIOPort  Port=2  Side=Left
  A2 : PMIOPort  Port=3  Side=Left
  A3 : PMIOPort  Port=4  Side=Left
  connections:
  B/RConn1 -- Chamber/LConn1 -- A3/RConn1 -- A2/RConn1 -- A1/RConn1

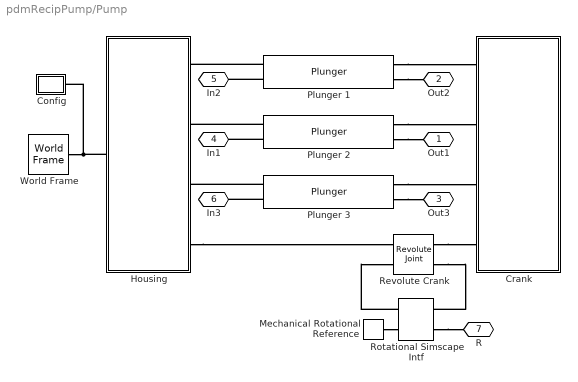
== system pdmRecipPump/Pump ==
  Config : Subsystem
  Crank : Subsystem  mask(Crankshaft){shaft_len=shaft_len_P, shaft_rad=shaft_rad_P, web_rad=web_rad_P, web_len=web_len_P, motor_shaft_rad=motor_shaft_rad_P, motor_shaft_len=motor_shaft_len_P, shaft_pos=shaft_pos_P, crank_rho=crank_rho_P, motor_shaft_clr=motor_shaft_clr_P, crank_clr=crank_clr_P, crank_opc=crank_opc_P}
      mask prompts: shaft_pos "Crankpin Axis Offset (m)"; crank_rho "Density (kg/m^3)"; motor_shaft_clr "Motor Shaft Color [RGB]"; crank_clr "Crank Color [RGB]"; crank_opc "Opacity (0-1)"
      mask help: Models pump crankshaft with three crankpins, each offset by 120 degrees from the crankshaft axis.
      mask DialogControl text_radius Prompt: Radius (m)
      mask DialogControl text_length Prompt: Length (m)
      mask DialogControl text_crankpin Prompt: Crankpin
      mask DialogControl text_web Prompt: Web
      mask DialogControl text_motor_shaft Prompt: Motor Shaft
      mask DialogControl cont_crank_vis Prompt: Crankshaft Visualization
      mask Display: image('sm_pump_triplex_Crank_IMAGE.png');
  Housing : Subsystem
      mask Display: image('sm_pump_triplex_Housing_IMAGE.png');
  Mechanical Rotational Reference : fl_lib/Mechanical/Rotational Elements/Mechanical Rotational Reference
  Plunger 1 : sm_pump_triplex_lib/Plunger  cyl_gap=cyl_gap_P  cyl_rad_out=cyl_rad_out_P  cyl_len=cyl_len_P  cyl_stroke=cyl_stroke_P  cyl_rad_in=0  cyl_xc_rev=0  cyl_frict_brkway_frc=cyl_frict_brkway_frc_P  cyl_frict_brkway_vel=cyl_frict_brkway_vel_P  cyl_frict_col_frc=cyl_frict_col_frc_P  cyl_frict_visc_coef=cyl_frict_visc_coef_P  cyl_rho=cyl_rho_P  cyl_clr=cyl_clr_P  cyl_opc=cyl_opc_P  plgB_len=plgB_len_P  plgB_rad=plgB_rad_P  stem_len=stem_len_P  stem_rad=stem_rad_P  pin_len=pin_len_P  pin_rad=pin_rad_P  cup_rad_out=cup_rad_out_P  cup_thk=cup_thk_P  cup_len=cup_len_P  cup_pinOffset=cup_pinOffset_P  cup_rad_in=0  plg_rho=plg_rho_P  plg_clr=plg_clr_P  plg_opc=plg_opc_P  conrod_len=conrod_len_P  conrod_web_widP=conrod_web_widP_P  conrod_web_widC=conrod_web_widC_P  conrod_web_offC=0  conrod_web_offP=0  conrod_web_len=0  conrod_web_xc=0  conrod_ringC_wid=conrod_ringC_wid_P  conrod_ringP_wid=conrod_ringP_wid_P  crank_shaft_rad=crank_shaft_rad_P  conrod_ringC_or=0  conrod_ringP_or=0  conrod_ringC_xc_rev=0  conrod_ringP_xc_rev=0  conrod_thk=conrod_thk_P  conrod_rho=conrod_rho_P  conrod_clr=conrod_clr_P  conrod_opc=conrod_opc_P  chkv_in_maxA=chkv_in_maxA_P  chkv_out_maxA=chkv_out_maxA_P  chkv_press_set_popup=Set in Mask  chkv_in_crkP=chkv_in_crkP_P  chkv_out_crkP=chkv_out_crkP_P  chkv_in_maxOpenP=chkv_in_maxOpenP_P  chkv_out_maxOpenP=chkv_out_maxOpenP_P  chkv_vis_popup=Off  chkv_vis_rad_in=chkv_vis_rad_in_P  chkv_vis_rad_out=chkv_vis_rad_out_P  chkv_vis_clr_in=chkv_vis_clr_in_P  chkv_vis_clr_out=chkv_vis_clr_out_P  leak_cyl_popup=On, Run Time  leak_cyl_area=leak_cyl2_area  block_in_popup=On, Run Time  block_in_factor=block_in_cyl2_factor  seal_leak_vis_len=seal_leak_vis_len_P  seal_leak_vis_rad=seal_leak_vis_rad_P  seal_leak_vis_clr=seal_leak_vis_clr_P  seal_leak_vis_opc=0  inlet_obstr_len=inlet_obstr_len_P  inlet_obstr_rad=inlet_obstr_rad_P  inlet_obstr_xc_rev=0  inlet_obstr_clr=inlet_obstr_clr_P  inlet_obstr_opc=1
  Plunger 2 : sm_pump_triplex_lib/Plunger  cyl_gap=cyl_gap_P  cyl_rad_out=cyl_rad_out_P  cyl_len=cyl_len_P  cyl_stroke=cyl_stroke_P  cyl_rad_in=0  cyl_xc_rev=0  cyl_frict_brkway_frc=cyl_frict_brkway_frc_P  cyl_frict_brkway_vel=cyl_frict_brkway_vel_P  cyl_frict_col_frc=cyl_frict_col_frc_P  cyl_frict_visc_coef=cyl_frict_visc_coef_P  cyl_rho=cyl_rho_P  cyl_clr=cyl_clr_P  cyl_opc=cyl_opc_P  plgB_len=plgB_len_P  plgB_rad=plgB_rad_P  stem_len=stem_len_P  stem_rad=stem_rad_P  pin_len=pin_len_P  pin_rad=pin_rad_P  cup_rad_out=cup_rad_out_P  cup_thk=cup_thk_P  cup_len=cup_len_P  cup_pinOffset=cup_pinOffset_P  cup_rad_in=0  plg_rho=plg_rho_P  plg_clr=plg_clr_P  plg_opc=plg_opc_P  conrod_len=conrod_len_P  conrod_web_widP=conrod_web_widP_P  conrod_web_widC=conrod_web_widC_P  conrod_web_offC=0  conrod_web_offP=0  conrod_web_len=0  conrod_web_xc=0  conrod_ringC_wid=conrod_ringC_wid_P  conrod_ringP_wid=conrod_ringP_wid_P  crank_shaft_rad=crank_shaft_rad_P  conrod_ringC_or=0  conrod_ringP_or=0  conrod_ringC_xc_rev=0  conrod_ringP_xc_rev=0  conrod_thk=conrod_thk_P  conrod_rho=conrod_rho_P  conrod_clr=conrod_clr_P  conrod_opc=conrod_opc_P  chkv_in_maxA=chkv_in_maxA_P  chkv_out_maxA=chkv_out_maxA_P  chkv_press_set_popup=Set in Mask  chkv_in_crkP=chkv_in_crkP_P  chkv_out_crkP=chkv_out_crkP_P  chkv_in_maxOpenP=chkv_in_maxOpenP_P  chkv_out_maxOpenP=chkv_out_maxOpenP_P  chkv_vis_popup=Off  chkv_vis_rad_in=chkv_vis_rad_in_P  chkv_vis_rad_out=chkv_vis_rad_out_P  chkv_vis_clr_in=chkv_vis_clr_in_P  chkv_vis_clr_out=chkv_vis_clr_out_P  leak_cyl_popup=Off  leak_cyl_area=leak_cyl2_area  block_in_popup=Off  block_in_factor=block_in_cyl2_factor  seal_leak_vis_len=seal_leak_vis_len_P  seal_leak_vis_rad=seal_leak_vis_rad_P  seal_leak_vis_clr=seal_leak_vis_clr_P  seal_leak_vis_opc=0  inlet_obstr_len=inlet_obstr_len_P  inlet_obstr_rad=inlet_obstr_rad_P  inlet_obstr_xc_rev=0  inlet_obstr_clr=inlet_obstr_clr_P  inlet_obstr_opc=1
  Plunger 3 : sm_pump_triplex_lib/Plunger  cyl_gap=cyl_gap_P  cyl_rad_out=cyl_rad_out_P  cyl_len=cyl_len_P  cyl_stroke=cyl_stroke_P  cyl_rad_in=0  cyl_xc_rev=0  cyl_frict_brkway_frc=cyl_frict_brkway_frc_P  cyl_frict_brkway_vel=cyl_frict_brkway_vel_P  cyl_frict_col_frc=cyl_frict_col_frc_P  cyl_frict_visc_coef=cyl_frict_visc_coef_P  cyl_rho=cyl_rho_P  cyl_clr=cyl_clr_P  cyl_opc=cyl_opc_P  plgB_len=plgB_len_P  plgB_rad=plgB_rad_P  stem_len=stem_len_P  stem_rad=stem_rad_P  pin_len=pin_len_P  pin_rad=pin_rad_P  cup_rad_out=cup_rad_out_P  cup_thk=cup_thk_P  cup_len=cup_len_P  cup_pinOffset=cup_pinOffset_P  cup_rad_in=0  plg_rho=plg_rho_P  plg_clr=plg_clr_P  plg_opc=plg_opc_P  conrod_len=conrod_len_P  conrod_web_widP=conrod_web_widP_P  conrod_web_widC=conrod_web_widC_P  conrod_web_offC=0  conrod_web_offP=0  conrod_web_len=0  conrod_web_xc=0  conrod_ringC_wid=conrod_ringC_wid_P  conrod_ringP_wid=conrod_ringP_wid_P  crank_shaft_rad=crank_shaft_rad_P  conrod_ringC_or=0  conrod_ringP_or=0  conrod_ringC_xc_rev=0  conrod_ringP_xc_rev=0  conrod_thk=conrod_thk_P  conrod_rho=conrod_rho_P  conrod_clr=conrod_clr_P  conrod_opc=conrod_opc_P  chkv_in_maxA=chkv_in_maxA_P  chkv_out_maxA=chkv_out_maxA_P  chkv_press_set_popup=Set in Mask  chkv_in_crkP=chkv_in_crkP_P  chkv_out_crkP=chkv_out_crkP_P  chkv_in_maxOpenP=chkv_in_maxOpenP_P  chkv_out_maxOpenP=chkv_out_maxOpenP_P  chkv_vis_popup=Off  chkv_vis_rad_in=chkv_vis_rad_in_P  chkv_vis_rad_out=chkv_vis_rad_out_P  chkv_vis_clr_in=chkv_vis_clr_in_P  chkv_vis_clr_out=chkv_vis_clr_out_P  leak_cyl_popup=Off  leak_cyl_area=leak_cyl3_area  block_in_popup=Off  block_in_factor=block_in_cyl3_factor  seal_leak_vis_len=seal_leak_vis_len_P  seal_leak_vis_rad=seal_leak_vis_rad_P  seal_leak_vis_clr=seal_leak_vis_clr_P  seal_leak_vis_opc=0  inlet_obstr_len=inlet_obstr_len_P  inlet_obstr_rad=inlet_obstr_rad_P  inlet_obstr_xc_rev=0  inlet_obstr_clr=inlet_obstr_clr_P  inlet_obstr_opc=1
  Revolute Crank : sm_lib/Joints/Revolute Joint  JointMode=Normal  CompositeWrenchDir=FollowerOnBase  CompositeWrenchFrame=BaseFrame  SenseConstraintForce=off  SenseConstraintTorque=off  SenseTotalForce=off  SenseTotalTorque=off  PositionTargetSpecify=off  PositionTargetPriority=High  PositionTargetValue=0  PositionTargetValueUnits=deg  VelocityTargetSpecify=off  VelocityTargetPriority=High  VelocityTargetValue=0  VelocityTargetValueUnits=deg/s  EquilibriumPosition=0  EquilibriumPositionUnits=deg  SpringStiffness=0  SpringStiffnessUnits=N*m/deg  DampingCoefficient=bearing_visc_frict_WKSP+bearing_fault_frict_WKSP  DampingCoefficientUnits=N*m/(deg/s)  LowerLimitSpecify=off  LowerLimitBound=-90  LowerLimitBoundUnits=deg  LowerLimitStiffness=1e4  LowerLimitStiffnessUnits=N*m/deg  LowerLimitDamping=10  LowerLimitDampingUnits=N*m/(deg/s)  LowerLimitTransitionRegionWidth=0.1  LowerLimitTransitionRegionWidthUnits=deg  UpperLimitSpecify=off  UpperLimitBound=90  UpperLimitBoundUnits=deg  UpperLimitStiffness=1e4  UpperLimitStiffnessUnits=N*m/deg  UpperLimitDamping=10  UpperLimitDampingUnits=N*m/(deg/s)  UpperLimitTransitionRegionWidth=0.1  UpperLimitTransitionRegionWidthUnits=deg  TorqueActuationMode=InputTorque  MotionActuationMode=ComputedMotion  SensePosition=off  SenseVelocity=on  SenseAcceleration=off  SenseTorqueForce=off  SenseLowerLimitTorqueForce=off  SenseUpperLimitTorqueForce=off
  Rotational Simscape Intf : Mech_Hydro_Elec_Multibody_Lib/Interfaces/Rotational Simscape Intf  SystemSampleTime=-1  VariantActivationTime=update diagram  EmptyChoice=off  PassThrough=off  PassThroughVariantControl=(default)  EmptyChoiceVariantControl=(default)  AllowFlexibleInterface=on  Latency=0  AutoFrameSizeCalculation=off
  World Frame : sm_lib/Frames and Transforms/World Frame
  Out1 : PMIOPort  Side=Right
  Out2 : PMIOPort  Port=2  Side=Right
  Out3 : PMIOPort  Port=3  Side=Right
  In1 : PMIOPort  Port=4  Side=Right
  In2 : PMIOPort  Port=5  Side=Right
  In3 : PMIOPort  Port=6  Side=Right
  R : PMIOPort  Port=7  Side=Left
  connections:
  Housing/LConn1 -- World Frame/RConn1 -- Config/RConn1
  Plunger 2/LConn1 -- Housing/RConn2
  Plunger 1/LConn2 -- In2/RConn1
  Plunger 1/RConn1 -- Crank/LConn1
  Plunger 2/RConn1 -- Crank/LConn2
  Plunger 3/LConn2 -- In3/RConn1
  Plunger 3/RConn2 -- Out3/RConn1
  Revolute Crank/RConn2 -- Rotational Simscape Intf/RConn1
  Plunger 1/LConn1 -- Housing/RConn1
  Plunger 2/LConn2 -- In1/RConn1
  Plunger 3/LConn1 -- Housing/RConn3
  Mechanical Rotational Reference/LConn1 -- Rotational Simscape Intf/LConn2
  Rotational Simscape Intf/LConn1 -- Revolute Crank/LConn2
  Housing/RConn4 -- Revolute Crank/LConn1
  Revolute Crank/RConn1 -- Crank/LConn4
  Plunger 1/RConn2 -- Out2/RConn1
  Plunger 2/RConn2 -- Out1/RConn1
  Plunger 3/RConn1 -- Crank/LConn3
  Rotational Simscape Intf/RConn2 -- R/RConn1

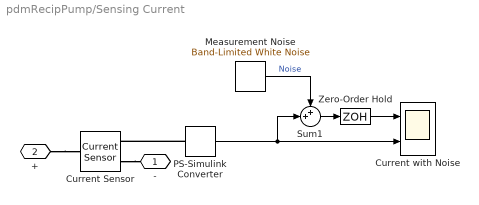
== system pdmRecipPump/Sensing Current ==
  Current Sensor : fl_lib/Electrical/Electrical Sensors/Current Sensor
  Current with Noise : Scope  NumInputPorts=2
      settings: ActiveDisplayYMinimum=-5.56656  ActiveDisplayYMaximum=49.76256  DataLoggingVariableName=ScopeData2
  Measurement Noise : simulink/Sources/Band-Limited White Noise  Cov=TRP_Par.Sensors.i.Np  Ts=TRP_Par.Sensors.i.Ts  seed=TRP_Par.Sensors.i.Seed+noise_seed_offset_WKSP
  PS-Simulink Converter : nesl_utility/PS-Simulink Converter  PhysicalDomain=network_engine_domain  SubClassName=ps_output  LeftPortType=input  RightPortType=output  PseudoPeriodic=off  Frequencies=[]  VectorFormat=1-D array  Unit=1  AffineConversion=off
  Sum1 : Sum  Inputs=++|
  Zero-Order Hold : ZeroOrderHold  SampleTime=TRP_Par.Sensors.i.Ts
  - : PMIOPort  Side=Right
  + : PMIOPort  Port=2  Side=Left
  wires:
  Measurement Noise/1 -> Sum1/1  "Noise"
  Sum1/1 -> Zero-Order Hold/1
  PS-Simulink Converter/1 -> Sum1/2, Current with Noise/2
  Zero-Order Hold/1 -> Current with Noise/1
  connections:
  PS-Simulink Converter/LConn1 -- Current Sensor/RConn1
  +/RConn1 -- Current Sensor/LConn1
  Current Sensor/RConn2 -- -/RConn1
